simulink model "Bloque_Maquina_Sinc_Modelo_NL"  (R2023a)
settings: Solver=VariableStepAuto  StartTime=0.0  StopTime=10.0  RelTol=1e-3
values from neighbouring files (symbols this model uses):
  k_l = m*g*l_cm + m_l*g*l_l    (= 9.80665)    [variables.m]
  r = 120    [variables.m]
undefined symbols (not defined in the file or in its folder): alpha_Cu, b_eq, Cts, J_eq, lambda, Ld, Lls, Lq, Pp, Rts, Ts_ref
settings Model: Creator=Renzo  LastModifiedBy=tobip

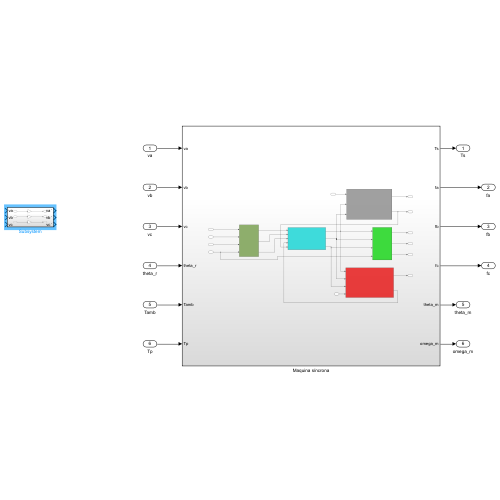
[thumbnail: Simulink's stored preview of the top-level diagram]
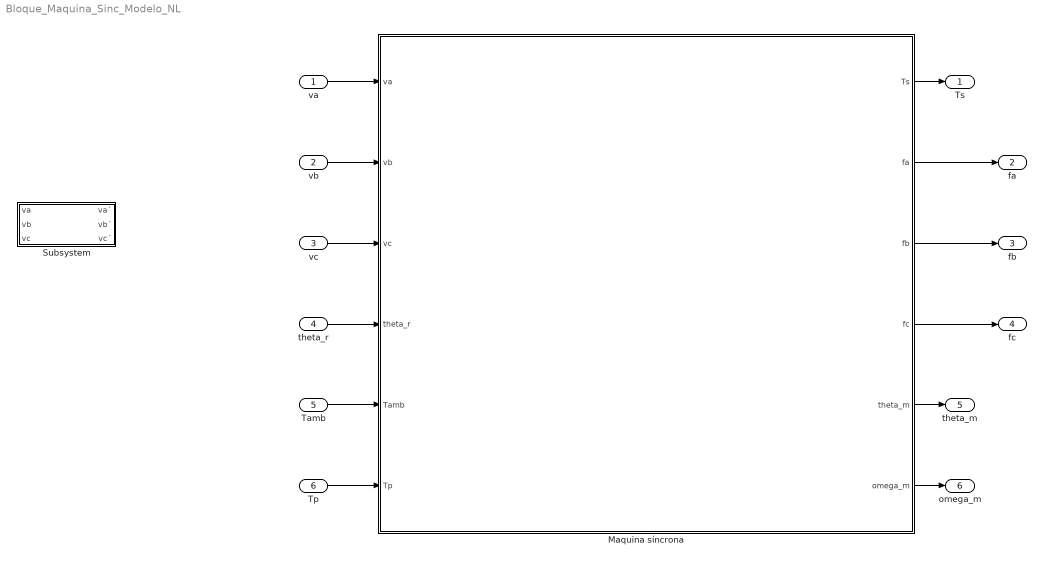
== system Bloque_Maquina_Sinc_Modelo_NL ==
  va : Inport
  vb : Inport  Port=2
  vc : Inport  Port=3
  theta_r : Inport  Port=4
  Tamb : Inport  Port=5
  Tp : Inport  Port=6
  Maquina síncrona : Subsystem
  Subsystem : Subsystem
  Ts : Outport
  fa : Outport  Port=2
  fb : Outport  Port=3
  fc : Outport  Port=4
  theta_m : Outport  Port=5
  omega_m : Outport  Port=6
  wires:
  va/1 -> Maquina síncrona/1(va)
  vb/1 -> Maquina síncrona/2(vb)
  vc/1 -> Maquina síncrona/3(vc)
  theta_r/1 -> Maquina síncrona/4(theta_r)
  Tamb/1 -> Maquina síncrona/5(Tamb)
  Tp/1 -> Maquina síncrona/6(Tp)
  Maquina síncrona/1(Ts) -> Ts/1
  Maquina síncrona/2(fa) -> fa/1
  Maquina síncrona/3(fb) -> fb/1
  Maquina síncrona/4(fc) -> fc/1
  Maquina síncrona/5(theta_m) -> theta_m/1
  Maquina síncrona/6(omega_m) -> omega_m/1

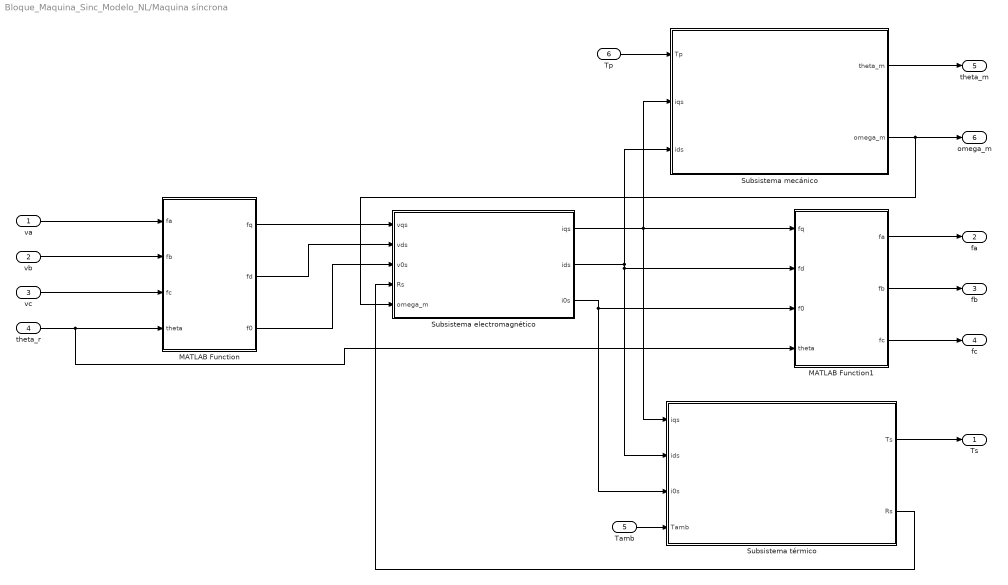
== system Bloque_Maquina_Sinc_Modelo_NL/Maquina síncrona ==
  va : Inport
  vb : Inport  Port=2
  vc : Inport  Port=3
  theta_r : Inport  Port=4
  Tamb : Inport  Port=5
  Tp : Inport  Port=6
  MATLAB Function : MATLAB Function  TreatAsAtomicUnit=on
  MATLAB Function1 : MATLAB Function  TreatAsAtomicUnit=on
  Subsistema electromagnético : Subsystem
  Subsistema mecánico : Subsystem
  Subsistema térmico : Subsystem
  Ts : Outport
  fa : Outport  Port=2
  fb : Outport  Port=3
  fc : Outport  Port=4
  theta_m : Outport  Port=5
  omega_m : Outport  Port=6
  wires:
  theta_r/1 -> MATLAB Function/4(theta), MATLAB Function1/4(theta)
  Subsistema mecánico/2(omega_m) -> omega_m/1, Subsistema electromagnético/5(omega_m)
  va/1 -> MATLAB Function/1(fa)
  vc/1 -> MATLAB Function/3(fc)
  Subsistema electromagnético/2(ids) -> Subsistema térmico/2(ids), MATLAB Function1/2(fd), Subsistema mecánico/3(ids)
  MATLAB Function/3(f0) -> Subsistema electromagnético/3(v0s)
  MATLAB Function/2(fd) -> Subsistema electromagnético/2(vds)
  Tp/1 -> Subsistema mecánico/1(Tp)
  Tamb/1 -> Subsistema térmico/4(Tamb)
  MATLAB Function/1(fq) -> Subsistema electromagnético/1(vqs)
  Subsistema electromagnético/3(i0s) -> MATLAB Function1/3(f0), Subsistema térmico/3(i0s)
  Subsistema electromagnético/1(iqs) -> MATLAB Function1/1(fq), Subsistema térmico/1(iqs), Subsistema mecánico/2(iqs)
  MATLAB Function1/2(fb) -> fb/1
  MATLAB Function1/1(fa) -> fa/1
  MATLAB Function1/3(fc) -> fc/1
  vb/1 -> MATLAB Function/2(fb)
  Subsistema térmico/2(Rs) -> Subsistema electromagnético/4(Rs)
  Subsistema térmico/1(Ts) -> Ts/1
  Subsistema mecánico/1(theta_m) -> theta_m/1

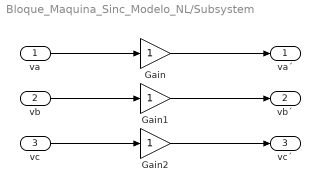
== system Bloque_Maquina_Sinc_Modelo_NL/Subsystem ==
  va : Inport
  vb : Inport  Port=2
  vc : Inport  Port=3
  Gain : Gain
  Gain1 : Gain
  Gain2 : Gain
  va´ : Outport
  vb´ : Outport  Port=2
  vc´ : Outport  Port=3
  wires:
  va/1 -> Gain/1
  Gain/1 -> va´/1
  vb/1 -> Gain1/1
  Gain1/1 -> vb´/1
  vc/1 -> Gain2/1
  Gain2/1 -> vc´/1

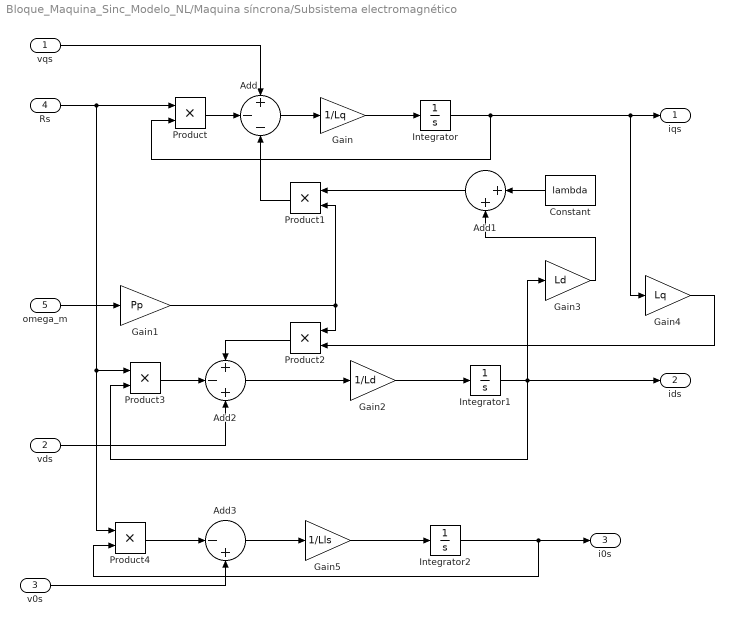
== system Bloque_Maquina_Sinc_Modelo_NL/Maquina síncrona/Subsistema electromagnético ==
  vqs : Inport
  vds : Inport  Port=2
  v0s : Inport  Port=3
  Rs : Inport  Port=4
  omega_m : Inport  Port=5
  Add : Sum  Inputs=+--
  Add1 : Sum  Inputs=|++
  Add2 : Sum  Inputs=+-+
  Add3 : Sum  Inputs=|-+
  Constant : Constant  Value=lambda
  Gain : Gain  Gain=1/Lq
  Gain1 : Gain  Gain=Pp
  Gain2 : Gain  Gain=1/Ld
  Gain3 : Gain  Gain=Ld
  Gain4 : Gain  Gain=Lq
  Gain5 : Gain  Gain=1/Lls
  Integrator : Integrator
  Integrator1 : Integrator
  Integrator2 : Integrator
  Product{,1..4} (5 alike) : Product
  iqs : Outport
  ids : Outport  Port=2
  i0s : Outport  Port=3
  wires:
  vqs/1 -> Add/1
  Gain/1 -> Integrator/1
  Add/1 -> Gain/1
  Integrator/1 -> Product/2, Gain4/1, iqs/1
  Product/1 -> Add/2
  Rs/1 -> Product/1, Product4/1, Product3/1
  Constant/1 -> Add1/1
  Add1/1 -> Product1/1
  Gain1/1 -> Product2/1, Product1/2
  Product1/1 -> Add/3
  omega_m/1 -> Gain1/1
  Product2/1 -> Add2/1
  vds/1 -> Add2/3
  Product3/1 -> Add2/2
  Add2/1 -> Gain2/1
  Gain2/1 -> Integrator1/1
  Integrator1/1 -> Gain3/1, ids/1, Product3/2
  Gain4/1 -> Product2/2
  Gain3/1 -> Add1/2
  v0s/1 -> Add3/2
  Product4/1 -> Add3/1
  Add3/1 -> Gain5/1
  Gain5/1 -> Integrator2/1
  Integrator2/1 -> Product4/2, i0s/1

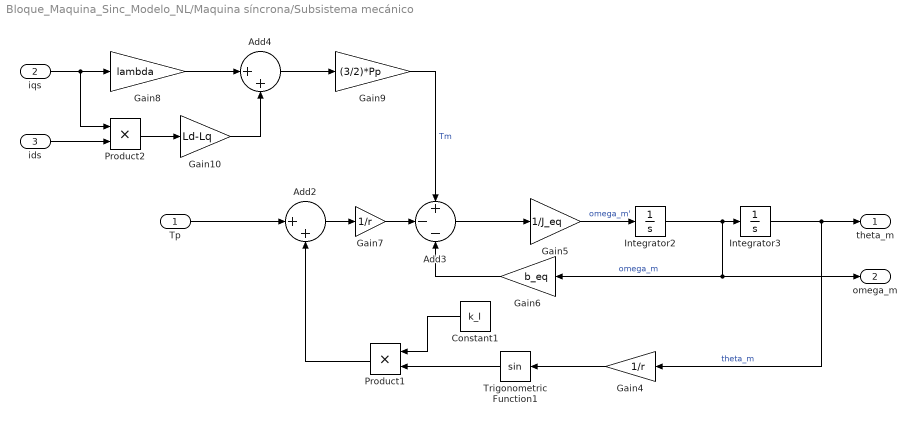
== system Bloque_Maquina_Sinc_Modelo_NL/Maquina síncrona/Subsistema mecánico ==
  Tp : Inport
  iqs : Inport  Port=2
  ids : Inport  Port=3
  Add2 : Sum  Inputs=|++
  Add3 : Sum  Inputs=+--
  Add4 : Sum  Inputs=|++
  Constant1 : Constant  Value=k_l
  Gain10 : Gain  Gain=Ld-Lq
  Gain4 : Gain  Gain=1/r
  Gain5 : Gain  Gain=1/J_eq
  Gain6 : Gain  Gain=b_eq
  Gain7 : Gain  Gain=1/r
  Gain8 : Gain  Gain=lambda
  Gain9 : Gain  Gain=(3/2)*Pp
  Integrator2 : Integrator
  Integrator3 : Integrator
  Product1 : Product
  Product2 : Product
  Trigonometric Function1 : Trigonometry
  theta_m : Outport
  omega_m : Outport  Port=2
  wires:
  Add2/1 -> Gain7/1
  Integrator2/1 -> omega_m/1, Gain6/1, Integrator3/1  "omega_m"
  Gain6/1 -> Add3/3
  Gain4/1 -> Trigonometric Function1/1
  Integrator3/1 -> theta_m/1, Gain4/1  "theta_m"
  iqs/1 -> Product2/1, Gain8/1
  Product1/1 -> Add2/2
  Add3/1 -> Gain5/1
  Gain5/1 -> Integrator2/1  "omega_m'"
  Constant1/1 -> Product1/1
  Tp/1 -> Add2/1
  Trigonometric Function1/1 -> Product1/2
  Gain8/1 -> Add4/1
  Gain7/1 -> Add3/2
  Add4/1 -> Gain9/1
  Gain9/1 -> Add3/1  "Tm"
  Product2/1 -> Gain10/1
  Gain10/1 -> Add4/2
  ids/1 -> Product2/2

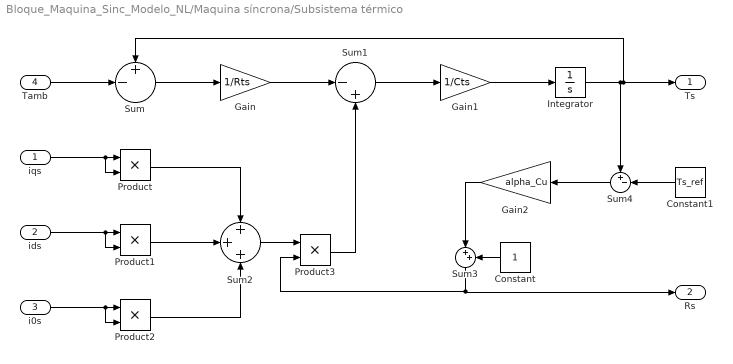
== system Bloque_Maquina_Sinc_Modelo_NL/Maquina síncrona/Subsistema térmico ==
  iqs : Inport
  ids : Inport  Port=2
  i0s : Inport  Port=3
  Tamb : Inport  Port=4
  Constant : Constant
  Constant1 : Constant  Value=Ts_ref
  Gain : Gain  Gain=1/Rts
  Gain1 : Gain  Gain=1/Cts
  Gain2 : Gain  Gain=alpha_Cu
  Integrator : Integrator
  Product{,1..3} (4 alike) : Product
  Sum : Sum  Inputs=+-|
  Sum1 : Sum  Inputs=|-+
  Sum2 : Sum  Inputs=+++
  Sum3 : Sum  Inputs=|++
  Sum4 : Sum  Inputs=+-|
  Ts : Outport
  Rs : Outport  Port=2
  wires:
  Tamb/1 -> Sum/2
  Gain/1 -> Sum1/1
  Sum/1 -> Gain/1
  Sum1/1 -> Gain1/1
  Gain1/1 -> Integrator/1
  Integrator/1 -> Ts/1, Sum/1, Sum4/1
  iqs/1 -> Product/2, Product/1
  ids/1 -> Product1/2, Product1/1
  i0s/1 -> Product2/2, Product2/1
  Product1/1 -> Sum2/2
  Product/1 -> Sum2/1
  Product2/1 -> Sum2/3
  Sum2/1 -> Product3/1
  Product3/1 -> Sum1/2
  Constant/1 -> Sum3/2
  Gain2/1 -> Sum3/1
  Constant1/1 -> Sum4/2
  Sum4/1 -> Gain2/1
  Sum3/1 -> Product3/2, Rs/1

== matlab function Bloque_Maquina_Sinc_Modelo_NL/Maquina síncrona/MATLAB Function1 ==
  data: fq input; fa output; fd input; f0 input; theta input; fb output; fc output
function [fa,fb,fc] = TI_Park(fq,fd,f0,theta)

f = (2/3)*[     cos(theta)              sin(theta)         1;
           cos(theta - (2*pi)/3)   sin(theta - (2*pi)/3)   1;
           cos(theta + (2*pi)/3)   sin(theta + (2*pi)/3)   1];

[fa;fb;fc] = f*[fq;fd;f0];

== matlab function Bloque_Maquina_Sinc_Modelo_NL/Maquina síncrona/MATLAB Function ==
  data: fa input; fq output; fb input; fc input; theta input; fd output; f0 output
function [fq,fd,f0] = TD_Park(fa,fb,fc,theta)

f = (2/3)*[cos(theta)  cos(theta - (2*pi)/3)   cos(theta + (2*pi)/3);
           sin(theta)  sin(theta - (2*pi)/3)   sin(theta + (2*pi)/3);
              1/2              1/2                     1/2         ];

[fq;fd;f0] = f*[fa;fb;fc];
